simulink model "lab2_simulink"  (R2017a)
settings: Solver=ode45  StartTime=0.0  StopTime=3  MaxStep=.001  RelTol=1e-3
values from neighbouring files (symbols this model uses):
  A = [-6 -25; 1 0]    [lab2.m]
  B = [25; 0]    [lab2.m]
  C = [1 0; 0 1]    [lab2.m]
  D = [0; 0]    [lab2.m]
settings Model: Creator=kg3  LastModifiedBy=kg3

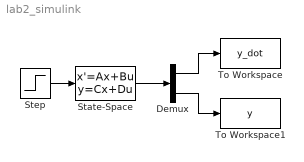
== system lab2_simulink ==
  Demux : Demux  Outputs=2
  State-Space : StateSpace  A=A  B=B  C=C  D=D  X0=0
  Step : Step  Time=0  SampleTime=0
  To Workspace : ToWorkspace  VariableName=y_dot  SaveFormat=Timeseries  SampleTime=-1
  To Workspace1 : ToWorkspace  VariableName=y  SaveFormat=Timeseries  SampleTime=-1
  wires:
  Step/1 -> State-Space/1
  State-Space/1 -> Demux/1
  Demux/2 -> To Workspace1/1
  Demux/1 -> To Workspace/1
